simulink model "Tractor_BURGERS_etrailer_v2_1_backup070824"  (R2023a)
settings: Solver=VariableStepAuto  StartTime=0.0  StopTime=tmax  FixedStep=dt  RelTol=1e-3  EnableMultiTasking=on
PreLoadFcn:
  | init_vehicle
  | SIMSCAPE_BE_driveline_etrailer_parameters
StartFcn:
  | tic
StopFcn:
  | toc
  | sim_stop_function
  | Etrailer_Simscape_MBM_plotting
undefined symbols (not defined in the file): brake_input, chassis_length, Diesel_density, Eff, end_val, energyCapacity, etrailer_ON, final_x, final_y, Floor, front_overhang, G_motor, initialSOC, InputSwitch, L_0f, LD, mass_trailer, massload, MaxTrqOut, pose_t0, RPM, sp_t, Std_Regen_Trq, steer_input, steer_path, steer_ratio, steer_sens, throttle_input, tire_param_drive, tire_param_steer, tire_param_trailer, tire_width, Torq, v_0, Voc, Vx, Vx_input, wheelbase, X, Y, Z
libraries: sm_lib x367, nesl_utility x282, fl_lib x20, sdl_lib x2, ee_lib x2, robotalgslib x1, simulink_extras x1, batteryecm_lib x1, BatteryEstimators x1, CommercialVehicleLibrary2G x1
(part 5 of 12)

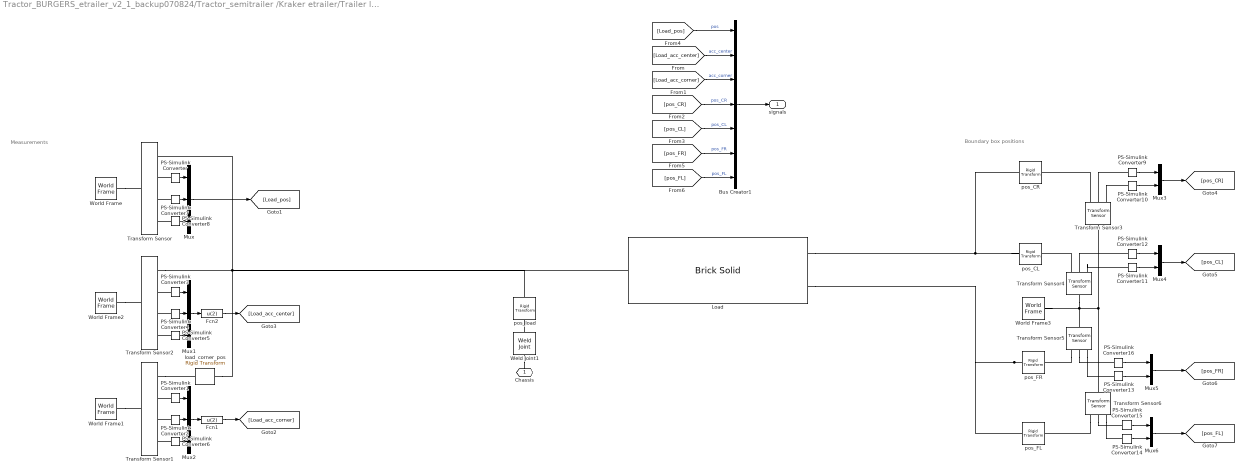
== system Tractor_BURGERS_etrailer_v2_1_backup070824/Tractor_semitrailer /Kraker etrailer/Trailer load front ==
  note: Boundary box positions
  note: Measurements
  Bus Creator1 : BusCreator  Inputs=7
  Fcn1 : Fcn  Expr=u(2)
  Fcn2 : Fcn  Expr=u(2)
  "Load " : sm_lib/Body Elements/Brick Solid  GraphicAmbientColor=[0.15 0.15 0.15 1.0]  BasedOnType=Density  BrickDimensions=[l_load w h]  BrickDimensionsUnits=m  CenterOfMass=[0 0 0]  CenterOfMassUnits=m  GraphicDiffuseColor=[1.0 1.0 0.2]  Density=1000  DensityUnits=kg/m^3  DoExposeReferenceFrame=on  GraphicEmissiveColor=[0.0 0.0 0.0 1.0]  ExportEntireGeometry=off  SerializedFrames=<Frames><Frame><Id>Frame1</Id><Value><Name>Boundary Center</Name><Origin><Source>GeometricFeature</Source><FeatureName>-x surface</FeatureName></Origin><PrimaryAxis><DefinedDirection>+Z</DefinedDirection><Source>ReferenceFrame</Source><SourceDirection>+Z</SourceDirection><FeatureName></FeatureName></PrimaryAxis><SecondaryAxis><DefinedDirection>+X</DefinedDirection><Source>ReferenceFrame</Source><SourceDirection>+X</SourceDirection><FeatureName></FeatureName></SecondaryAxis></Value></Frame><Frame><Id>Frame2</Id><Value><Name>Boundary Front </Name><Origin><Source>GeometricFeature</Source><FeatureName>+x surface</FeatureName></Origin><PrimaryAxis><DefinedDirection>+Z</DefinedDirection><Source>ReferenceFrame</Source><SourceDirection>+Z</SourceDirection><FeatureName></FeatureName></PrimaryAxis><SecondaryAxis><DefinedDirection>+X</DefinedDirection><Source>ReferenceFrame</Source><SourceDirection>+X</SourceDirection><FeatureName></FeatureName></SecondaryAxis></Value></Frame></Frames>  MarkerShape=Sphere  MarkerSize=10  GraphicType=FromGeometry  InertiaType=Custom  Mass=mass_load  MassUnits=kg  MomentsOfInertia=[Ixx Iyy Izz]  MomentsOfInertiaUnits=kg*m^2  GraphicOpacity=0.5  ProductsOfInertia=[0 0 0]  ProductsOfInertiaUnits=kg*m^2  GraphicShininess=75  GraphicSpecularColor=[0.5 0.5 0.5 1.0]  GraphicVisPropType=SimpleVisualProperties
  Mux : Mux  Inputs=3
  Mux1 : Mux  Inputs=3
  Mux2 : Mux  Inputs=3
  Mux{3..6} (4 alike) : Mux  Inputs=2
  PS-Simulink Converter{,7..16} (11 alike) : nesl_utility/PS-Simulink Converter  PhysicalDomain=network_engine_domain  SubClassName=ps_output  LeftPortType=input  RightPortType=output  PseudoPeriodic=off  Frequencies=[]  VectorFormat=1-D array  Unit=inherit  AffineConversion=off
  PS-Simulink Converter{1..6} (6 alike) : nesl_utility/PS-Simulink Converter  PhysicalDomain=network_engine_domain  SubClassName=ps_output  LeftPortType=input  RightPortType=output  PseudoPeriodic=off  Frequencies=[]  VectorFormat=1-D array  Unit=m/s^2  AffineConversion=off
  Transform Sensor : sm_lib/Frames and Transforms/Transform Sensor  MeasurementFrame=World  RotationSequence=XYX  SenseAngle=off  SenseAxis=off  SenseQ=off  SenseR=off  SenseRotationSequence=off  SenseOmegaX=off  SenseOmegaY=off  SenseOmegaZ=off  SenseQDot=off  SenseRDot=off  SenseRotationSequenceDot=off  SenseAlphaX=off  SenseAlphaY=off  SenseAlphaZ=off  SenseQDDot=off  SenseRDDot=off  SenseX=on  SenseY=on  SenseZ=on  SenseRad=off  SenseAzim=off  SenseDist=off  SenseInc=off  SenseXDot=off  SenseYDot=off  SenseZDot=off  SenseRadDot=off  SenseAzimDot=off  SenseDistDot=off  SenseIncDot=off  SenseXDDot=off  SenseYDDot=off  SenseZDDot=off  SenseRadDDot=off  SenseAzimDDot=off  SenseDistDDot=off  SenseIncDDot=off
  Transform Sensor1 : sm_lib/Frames and Transforms/Transform Sensor  MeasurementFrame=NonRotatingFollower  RotationSequence=XYX  SenseAngle=off  SenseAxis=off  SenseQ=off  SenseR=off  SenseRotationSequence=off  SenseOmegaX=off  SenseOmegaY=off  SenseOmegaZ=off  SenseQDot=off  SenseRDot=off  SenseRotationSequenceDot=off  SenseAlphaX=off  SenseAlphaY=off  SenseAlphaZ=off  SenseQDDot=off  SenseRDDot=off  SenseX=off  SenseY=off  SenseZ=off  SenseRad=off  SenseAzim=off  SenseDist=off  SenseInc=off  SenseXDot=off  SenseYDot=off  SenseZDot=off  SenseRadDot=off  SenseAzimDot=off  SenseDistDot=off  SenseIncDot=off  SenseXDDot=on  SenseYDDot=on  SenseZDDot=on  SenseRadDDot=off  SenseAzimDDot=off  SenseDistDDot=off  SenseIncDDot=off
  Transform Sensor2 : sm_lib/Frames and Transforms/Transform Sensor  MeasurementFrame=NonRotatingFollower  RotationSequence=XYX  SenseAngle=off  SenseAxis=off  SenseQ=off  SenseR=off  SenseRotationSequence=off  SenseOmegaX=off  SenseOmegaY=off  SenseOmegaZ=off  SenseQDot=off  SenseRDot=off  SenseRotationSequenceDot=off  SenseAlphaX=off  SenseAlphaY=off  SenseAlphaZ=off  SenseQDDot=off  SenseRDDot=off  SenseX=off  SenseY=off  SenseZ=off  SenseRad=off  SenseAzim=off  SenseDist=off  SenseInc=off  SenseXDot=off  SenseYDot=off  SenseZDot=off  SenseRadDot=off  SenseAzimDot=off  SenseDistDot=off  SenseIncDot=off  SenseXDDot=on  SenseYDDot=on  SenseZDDot=on  SenseRadDDot=off  SenseAzimDDot=off  SenseDistDDot=off  SenseIncDDot=off
  Transform Sensor{3..6} (4 alike) : sm_lib/Frames and Transforms/Transform Sensor  MeasurementFrame=World  RotationSequence=XYX  SenseAngle=off  SenseAxis=off  SenseQ=off  SenseR=off  SenseRotationSequence=off  SenseOmegaX=off  SenseOmegaY=off  SenseOmegaZ=off  SenseQDot=off  SenseRDot=off  SenseRotationSequenceDot=off  SenseAlphaX=off  SenseAlphaY=off  SenseAlphaZ=off  SenseQDDot=off  SenseRDDot=off  SenseX=on  SenseY=on  SenseZ=off  SenseRad=off  SenseAzim=off  SenseDist=off  SenseInc=off  SenseXDot=off  SenseYDot=off  SenseZDot=off  SenseRadDot=off  SenseAzimDot=off  SenseDistDot=off  SenseIncDot=off  SenseXDDot=off  SenseYDDot=off  SenseZDDot=off  SenseRadDDot=off  SenseAzimDDot=off  SenseDistDDot=off  SenseIncDDot=off
  Weld Joint1 : sm_lib/Joints/Weld Joint  JointMode=Normal  SenseConstraintForce=off  SenseConstraintForceX=off  SenseConstraintForceY=off  SenseConstraintForceZ=off  SenseConstraintTorque=off  SenseConstraintTorqueX=off  SenseConstraintTorqueY=off  SenseConstraintTorqueZ=off  SenseTotalForce=off  SenseTotalForceX=off  SenseTotalForceY=off  SenseTotalForceZ=off  SenseTotalTorque=off  SenseTotalTorqueX=off  SenseTotalTorqueY=off  SenseTotalTorqueZ=off  CompositeWrenchDir=FollowerOnBase  CompositeWrenchFrame=BaseFrame
  World Frame{,1..3} (4 alike) : sm_lib/Frames and Transforms/World Frame
  load_corner_pos : sm_lib/Frames and Transforms/Rigid Transform  TranslationMethod=Cartesian  TranslationStandardOffset=0  TranslationStandardOffsetUnits=m  TranslationStandardAxis=+Z  TranslationCartesianOffset=[(-0.5*l_load) 0 0]  TranslationCartesianOffsetUnits=m  TranslationROffset=0  TranslationROffsetUnits=m  TranslationZOffset=0  TranslationZOffsetUnits=m  TranslationThetaOffset=0  TranslationThetaOffsetUnits=deg  RotationMethod=None  RotationAngleUnits=deg  RotationStandardAxis=+Z  RotationAngle=0.0  RotationArbitraryAxis=[0 0 1]  FollAlignAxisA=+X  BaseAlignAxisA=+Y  FollAlignAxisB=+Y  BaseAlignAxisB=+Z  RotationSequenceAxes=FollowerAxes  RotationSequence=XYX  RotationSequenceAngles=[0 0 0]  RotationSequenceAnglesUnits=deg  RotationMatrix=[1 0 0; 0 1 0; 0 0 1]  Quaternion=[1 0 0 0]
  pos_CL : sm_lib/Frames and Transforms/Rigid Transform  TranslationMethod=Cartesian  TranslationStandardOffset=0  TranslationStandardOffsetUnits=m  TranslationStandardAxis=+Z  TranslationCartesianOffset=[0 w/2 -h/2]  TranslationCartesianOffsetUnits=m  TranslationROffset=0  TranslationROffsetUnits=m  TranslationZOffset=0  TranslationZOffsetUnits=m  TranslationThetaOffset=0  TranslationThetaOffsetUnits=deg  RotationMethod=None  RotationAngleUnits=deg  RotationStandardAxis=+Z  RotationAngle=0.0  RotationArbitraryAxis=[0 0 1]  FollAlignAxisA=+X  BaseAlignAxisA=+Y  FollAlignAxisB=+Y  BaseAlignAxisB=+Z  RotationSequenceAxes=FollowerAxes  RotationSequence=XYX  RotationSequenceAngles=[0 0 0]  RotationSequenceAnglesUnits=deg  RotationMatrix=[1 0 0; 0 1 0; 0 0 1]  Quaternion=[1 0 0 0]
  pos_CR : sm_lib/Frames and Transforms/Rigid Transform  TranslationMethod=Cartesian  TranslationStandardOffset=0  TranslationStandardOffsetUnits=m  TranslationStandardAxis=+Z  TranslationCartesianOffset=[0 -w/2 -h/2]  TranslationCartesianOffsetUnits=m  TranslationROffset=0  TranslationROffsetUnits=m  TranslationZOffset=0  TranslationZOffsetUnits=m  TranslationThetaOffset=0  TranslationThetaOffsetUnits=deg  RotationMethod=None  RotationAngleUnits=deg  RotationStandardAxis=+Z  RotationAngle=0.0  RotationArbitraryAxis=[0 0 1]  FollAlignAxisA=+X  BaseAlignAxisA=+Y  FollAlignAxisB=+Y  BaseAlignAxisB=+Z  RotationSequenceAxes=FollowerAxes  RotationSequence=XYX  RotationSequenceAngles=[0 0 0]  RotationSequenceAnglesUnits=deg  RotationMatrix=[1 0 0; 0 1 0; 0 0 1]  Quaternion=[1 0 0 0]
  pos_FL : sm_lib/Frames and Transforms/Rigid Transform  TranslationMethod=Cartesian  TranslationStandardOffset=0  TranslationStandardOffsetUnits=m  TranslationStandardAxis=+Z  TranslationCartesianOffset=[0 w/2 -h/2]  TranslationCartesianOffsetUnits=m  TranslationROffset=0  TranslationROffsetUnits=m  TranslationZOffset=0  TranslationZOffsetUnits=m  TranslationThetaOffset=0  TranslationThetaOffsetUnits=deg  RotationMethod=None  RotationAngleUnits=deg  RotationStandardAxis=+Z  RotationAngle=0.0  RotationArbitraryAxis=[0 0 1]  FollAlignAxisA=+X  BaseAlignAxisA=+Y  FollAlignAxisB=+Y  BaseAlignAxisB=+Z  RotationSequenceAxes=FollowerAxes  RotationSequence=XYX  RotationSequenceAngles=[0 0 0]  RotationSequenceAnglesUnits=deg  RotationMatrix=[1 0 0; 0 1 0; 0 0 1]  Quaternion=[1 0 0 0]
  pos_FR : sm_lib/Frames and Transforms/Rigid Transform  TranslationMethod=Cartesian  TranslationStandardOffset=0  TranslationStandardOffsetUnits=m  TranslationStandardAxis=+Z  TranslationCartesianOffset=[0 -w/2 -h/2]  TranslationCartesianOffsetUnits=m  TranslationROffset=0  TranslationROffsetUnits=m  TranslationZOffset=0  TranslationZOffsetUnits=m  TranslationThetaOffset=0  TranslationThetaOffsetUnits=deg  RotationMethod=None  RotationAngleUnits=deg  RotationStandardAxis=+Z  RotationAngle=0.0  RotationArbitraryAxis=[0 0 1]  FollAlignAxisA=+X  BaseAlignAxisA=+Y  FollAlignAxisB=+Y  BaseAlignAxisB=+Z  RotationSequenceAxes=FollowerAxes  RotationSequence=XYX  RotationSequenceAngles=[0 0 0]  RotationSequenceAnglesUnits=deg  RotationMatrix=[1 0 0; 0 1 0; 0 0 1]  Quaternion=[1 0 0 0]
  pos_load : sm_lib/Frames and Transforms/Rigid Transform  TranslationMethod=Cartesian  TranslationStandardOffset=0  TranslationStandardOffsetUnits=m  TranslationStandardAxis=+Z  TranslationCartesianOffset=[-xcg1+xload 0 zcg+0.1]  TranslationCartesianOffsetUnits=m  TranslationROffset=0  TranslationROffsetUnits=m  TranslationZOffset=0  TranslationZOffsetUnits=m  TranslationThetaOffset=0  TranslationThetaOffsetUnits=deg  RotationMethod=None  RotationAngleUnits=deg  RotationStandardAxis=+Z  RotationAngle=0.0  RotationArbitraryAxis=[0 0 1]  FollAlignAxisA=+X  BaseAlignAxisA=+Y  FollAlignAxisB=+Y  BaseAlignAxisB=+Z  RotationSequenceAxes=FollowerAxes  RotationSequence=XYX  RotationSequenceAngles=[0 0 0]  RotationSequenceAnglesUnits=deg  RotationMatrix=[1 0 0; 0 1 0; 0 0 1]  Quaternion=[1 0 0 0]
  Chassis : PMIOPort  Side=Left
  signals : Outport
  wires:
  [Load_acc_corner] -> Bus Creator1/3  "acc_corner"
  PS-Simulink Converter1/1 -> Mux2/1
  Mux2/1 -> Fcn1/1
  PS-Simulink Converter6/1 -> Mux2/3
  Fcn1/1 -> [Load_acc_corner]
  PS-Simulink Converter2/1 -> Mux2/2
  [Load_pos] -> Bus Creator1/1  "pos"
  Bus Creator1/1 -> signals/1
  [Load_acc_center] -> Bus Creator1/2  "acc_center"
  PS-Simulink Converter4/1 -> Mux1/2
  Fcn2/1 -> [Load_acc_center]
  PS-Simulink Converter5/1 -> Mux1/3
  Mux/1 -> [Load_pos]
  Mux1/1 -> Fcn2/1
  PS-Simulink Converter3/1 -> Mux1/1
  PS-Simulink Converter8/1 -> Mux/3
  PS-Simulink Converter/1 -> Mux/1
  PS-Simulink Converter7/1 -> Mux/2
  PS-Simulink Converter9/1 -> Mux3/1
  PS-Simulink Converter10/1 -> Mux3/2
  PS-Simulink Converter11/1 -> Mux4/2
  PS-Simulink Converter12/1 -> Mux4/1
  Mux3/1 -> [pos_CR]
  Mux4/1 -> [pos_CL]
  Mux5/1 -> [pos_FR]
  PS-Simulink Converter14/1 -> Mux6/2
  PS-Simulink Converter15/1 -> Mux6/1
  Mux6/1 -> [pos_FL]
  PS-Simulink Converter16/1 -> Mux5/1
  PS-Simulink Converter13/1 -> Mux5/2
  [pos_CR] -> Bus Creator1/4  "pos_CR"
  [pos_FR] -> Bus Creator1/6  "pos_FR"
  [pos_CL] -> Bus Creator1/5  "pos_CL"
  [pos_FL] -> Bus Creator1/7  "pos_FL"
  connections:
  Transform Sensor1/RConn1 -- load_corner_pos/RConn1
  PS-Simulink Converter2/LConn1 -- Transform Sensor1/RConn3
  PS-Simulink Converter1/LConn1 -- Transform Sensor1/RConn2
  PS-Simulink Converter6/LConn1 -- Transform Sensor1/RConn4
  World Frame1/RConn1 -- Transform Sensor1/LConn1
  Weld Joint1/LConn1 -- Chassis/RConn1
  Weld Joint1/RConn1 -- pos_load/LConn1
  World Frame2/RConn1 -- Transform Sensor2/LConn1
  PS-Simulink Converter/LConn1 -- Transform Sensor/RConn2
  PS-Simulink Converter5/LConn1 -- Transform Sensor2/RConn4
  PS-Simulink Converter3/LConn1 -- Transform Sensor2/RConn2
  World Frame/RConn1 -- Transform Sensor/LConn1
  PS-Simulink Converter4/LConn1 -- Transform Sensor2/RConn3
  PS-Simulink Converter7/LConn1 -- Transform Sensor/RConn3
  PS-Simulink Converter8/LConn1 -- Transform Sensor/RConn4
  load_corner_pos/LConn1 -- Transform Sensor/RConn1 -- Transform Sensor2/RConn1 -- pos_load/RConn1 -- "Load "/RConn1
  pos_CL/LConn1 -- pos_CR/LConn1 -- "Load "/LConn1
  pos_FR/LConn1 -- "Load "/LConn2 -- pos_FL/LConn1
  World Frame3/RConn1 -- Transform Sensor5/LConn1 -- Transform Sensor4/LConn1 -- Transform Sensor3/LConn1 -- Transform Sensor6/LConn1
  Transform Sensor3/RConn1 -- pos_CR/RConn1
  Transform Sensor3/RConn2 -- PS-Simulink Converter9/LConn1
  Transform Sensor3/RConn3 -- PS-Simulink Converter10/LConn1
  Transform Sensor4/RConn1 -- pos_CL/RConn1
  Transform Sensor4/RConn2 -- PS-Simulink Converter12/LConn1
  Transform Sensor4/RConn3 -- PS-Simulink Converter11/LConn1
  Transform Sensor6/RConn2 -- PS-Simulink Converter15/LConn1
  Transform Sensor5/RConn3 -- PS-Simulink Converter13/LConn1
  Transform Sensor6/RConn1 -- pos_FL/RConn1
  Transform Sensor5/RConn2 -- PS-Simulink Converter16/LConn1
  Transform Sensor6/RConn3 -- PS-Simulink Converter14/LConn1
  Transform Sensor5/RConn1 -- pos_FR/RConn1

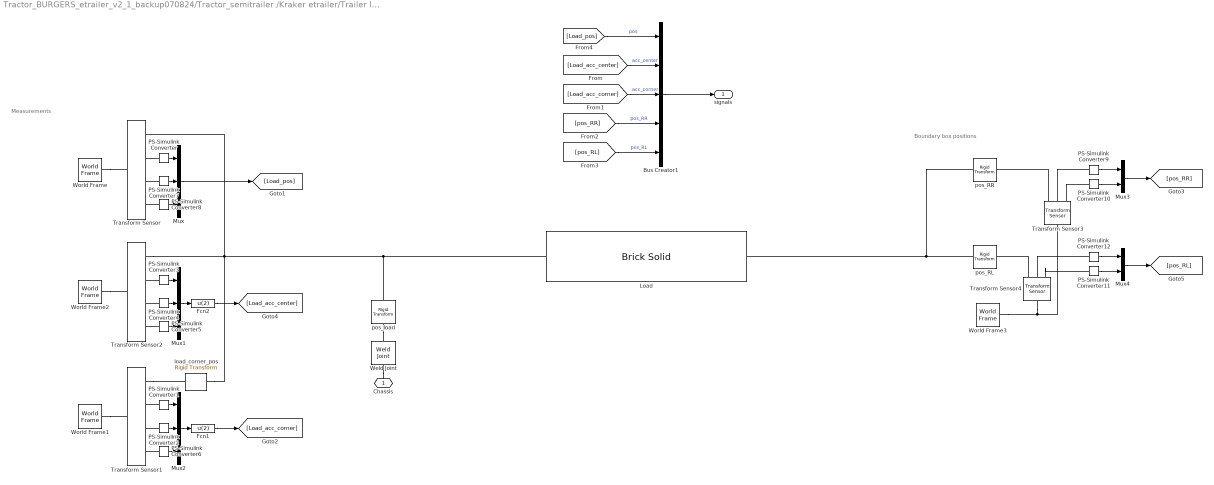
== system Tractor_BURGERS_etrailer_v2_1_backup070824/Tractor_semitrailer /Kraker etrailer/Trailer load rear ==
  note: Measurements
  note: Boundary box positions
  Bus Creator1 : BusCreator  Inputs=5
  Fcn1 : Fcn  Expr=u(2)
  Fcn2 : Fcn  Expr=u(2)
  "Load " : sm_lib/Body Elements/Brick Solid  GraphicAmbientColor=[0.15 0.15 0.15 1.0]  BasedOnType=Density  BrickDimensions=[l_load2 w h]  BrickDimensionsUnits=m  CenterOfMass=[0 0 0]  CenterOfMassUnits=m  GraphicDiffuseColor=[1.0 1.0 0.2]  Density=1000  DensityUnits=kg/m^3  DoExposeReferenceFrame=on  GraphicEmissiveColor=[0.0 0.0 0.0 1.0]  ExportEntireGeometry=off  SerializedFrames=<Frames><Frame><Id>Frame1</Id><Value><Name>Boundary rear </Name><Origin><Source>GeometricFeature</Source><FeatureName>-x surface</FeatureName></Origin><PrimaryAxis><DefinedDirection>+Z</DefinedDirection><Source>ReferenceFrame</Source><SourceDirection>+Z</SourceDirection><FeatureName></FeatureName></PrimaryAxis><SecondaryAxis><DefinedDirection>+X</DefinedDirection><Source>ReferenceFrame</Source><SourceDirection>+X</SourceDirection><FeatureName></FeatureName></SecondaryAxis></Value></Frame></Frames>  MarkerShape=Sphere  MarkerSize=10  GraphicType=FromGeometry  InertiaType=Custom  Mass=mass_load  MassUnits=kg  MomentsOfInertia=[Ixx Iyy Izz]  MomentsOfInertiaUnits=kg*m^2  GraphicOpacity=0.5  ProductsOfInertia=[0 0 0]  ProductsOfInertiaUnits=kg*m^2  GraphicShininess=75  GraphicSpecularColor=[0.5 0.5 0.5 1.0]  GraphicVisPropType=SimpleVisualProperties
  Mux : Mux  Inputs=3
  Mux1 : Mux  Inputs=3
  Mux2 : Mux  Inputs=3
  Mux3 : Mux  Inputs=2
  Mux4 : Mux  Inputs=2
  PS-Simulink Converter{,7..12} (7 alike) : nesl_utility/PS-Simulink Converter  PhysicalDomain=network_engine_domain  SubClassName=ps_output  LeftPortType=input  RightPortType=output  PseudoPeriodic=off  Frequencies=[]  VectorFormat=1-D array  Unit=inherit  AffineConversion=off
  PS-Simulink Converter{1..6} (6 alike) : nesl_utility/PS-Simulink Converter  PhysicalDomain=network_engine_domain  SubClassName=ps_output  LeftPortType=input  RightPortType=output  PseudoPeriodic=off  Frequencies=[]  VectorFormat=1-D array  Unit=m/s^2  AffineConversion=off
  Transform Sensor : sm_lib/Frames and Transforms/Transform Sensor  MeasurementFrame=World  RotationSequence=XYX  SenseAngle=off  SenseAxis=off  SenseQ=off  SenseR=off  SenseRotationSequence=off  SenseOmegaX=off  SenseOmegaY=off  SenseOmegaZ=off  SenseQDot=off  SenseRDot=off  SenseRotationSequenceDot=off  SenseAlphaX=off  SenseAlphaY=off  SenseAlphaZ=off  SenseQDDot=off  SenseRDDot=off  SenseX=on  SenseY=on  SenseZ=on  SenseRad=off  SenseAzim=off  SenseDist=off  SenseInc=off  SenseXDot=off  SenseYDot=off  SenseZDot=off  SenseRadDot=off  SenseAzimDot=off  SenseDistDot=off  SenseIncDot=off  SenseXDDot=off  SenseYDDot=off  SenseZDDot=off  SenseRadDDot=off  SenseAzimDDot=off  SenseDistDDot=off  SenseIncDDot=off
  Transform Sensor1 : sm_lib/Frames and Transforms/Transform Sensor  MeasurementFrame=NonRotatingFollower  RotationSequence=XYX  SenseAngle=off  SenseAxis=off  SenseQ=off  SenseR=off  SenseRotationSequence=off  SenseOmegaX=off  SenseOmegaY=off  SenseOmegaZ=off  SenseQDot=off  SenseRDot=off  SenseRotationSequenceDot=off  SenseAlphaX=off  SenseAlphaY=off  SenseAlphaZ=off  SenseQDDot=off  SenseRDDot=off  SenseX=off  SenseY=off  SenseZ=off  SenseRad=off  SenseAzim=off  SenseDist=off  SenseInc=off  SenseXDot=off  SenseYDot=off  SenseZDot=off  SenseRadDot=off  SenseAzimDot=off  SenseDistDot=off  SenseIncDot=off  SenseXDDot=on  SenseYDDot=on  SenseZDDot=on  SenseRadDDot=off  SenseAzimDDot=off  SenseDistDDot=off  SenseIncDDot=off
  Transform Sensor2 : sm_lib/Frames and Transforms/Transform Sensor  MeasurementFrame=NonRotatingFollower  RotationSequence=XYX  SenseAngle=off  SenseAxis=off  SenseQ=off  SenseR=off  SenseRotationSequence=off  SenseOmegaX=off  SenseOmegaY=off  SenseOmegaZ=off  SenseQDot=off  SenseRDot=off  SenseRotationSequenceDot=off  SenseAlphaX=off  SenseAlphaY=off  SenseAlphaZ=off  SenseQDDot=off  SenseRDDot=off  SenseX=off  SenseY=off  SenseZ=off  SenseRad=off  SenseAzim=off  SenseDist=off  SenseInc=off  SenseXDot=off  SenseYDot=off  SenseZDot=off  SenseRadDot=off  SenseAzimDot=off  SenseDistDot=off  SenseIncDot=off  SenseXDDot=on  SenseYDDot=on  SenseZDDot=on  SenseRadDDot=off  SenseAzimDDot=off  SenseDistDDot=off  SenseIncDDot=off
  Transform Sensor3 : sm_lib/Frames and Transforms/Transform Sensor  MeasurementFrame=World  RotationSequence=XYX  SenseAngle=off  SenseAxis=off  SenseQ=off  SenseR=off  SenseRotationSequence=off  SenseOmegaX=off  SenseOmegaY=off  SenseOmegaZ=off  SenseQDot=off  SenseRDot=off  SenseRotationSequenceDot=off  SenseAlphaX=off  SenseAlphaY=off  SenseAlphaZ=off  SenseQDDot=off  SenseRDDot=off  SenseX=on  SenseY=on  SenseZ=off  SenseRad=off  SenseAzim=off  SenseDist=off  SenseInc=off  SenseXDot=off  SenseYDot=off  SenseZDot=off  SenseRadDot=off  SenseAzimDot=off  SenseDistDot=off  SenseIncDot=off  SenseXDDot=off  SenseYDDot=off  SenseZDDot=off  SenseRadDDot=off  SenseAzimDDot=off  SenseDistDDot=off  SenseIncDDot=off
  Transform Sensor4 : sm_lib/Frames and Transforms/Transform Sensor  MeasurementFrame=World  RotationSequence=XYX  SenseAngle=off  SenseAxis=off  SenseQ=off  SenseR=off  SenseRotationSequence=off  SenseOmegaX=off  SenseOmegaY=off  SenseOmegaZ=off  SenseQDot=off  SenseRDot=off  SenseRotationSequenceDot=off  SenseAlphaX=off  SenseAlphaY=off  SenseAlphaZ=off  SenseQDDot=off  SenseRDDot=off  SenseX=on  SenseY=on  SenseZ=off  SenseRad=off  SenseAzim=off  SenseDist=off  SenseInc=off  SenseXDot=off  SenseYDot=off  SenseZDot=off  SenseRadDot=off  SenseAzimDot=off  SenseDistDot=off  SenseIncDot=off  SenseXDDot=off  SenseYDDot=off  SenseZDDot=off  SenseRadDDot=off  SenseAzimDDot=off  SenseDistDDot=off  SenseIncDDot=off
  Weld Joint : sm_lib/Joints/Weld Joint  JointMode=Normal  SenseConstraintForce=off  SenseConstraintForceX=off  SenseConstraintForceY=off  SenseConstraintForceZ=off  SenseConstraintTorque=off  SenseConstraintTorqueX=off  SenseConstraintTorqueY=off  SenseConstraintTorqueZ=off  SenseTotalForce=off  SenseTotalForceX=off  SenseTotalForceY=off  SenseTotalForceZ=off  SenseTotalTorque=off  SenseTotalTorqueX=off  SenseTotalTorqueY=off  SenseTotalTorqueZ=off  CompositeWrenchDir=FollowerOnBase  CompositeWrenchFrame=BaseFrame
  World Frame{,1..3} (4 alike) : sm_lib/Frames and Transforms/World Frame
  load_corner_pos : sm_lib/Frames and Transforms/Rigid Transform  TranslationMethod=Cartesian  TranslationStandardOffset=0  TranslationStandardOffsetUnits=m  TranslationStandardAxis=+Z  TranslationCartesianOffset=[(-0.5*l_load) 0 0]  TranslationCartesianOffsetUnits=m  TranslationROffset=0  TranslationROffsetUnits=m  TranslationZOffset=0  TranslationZOffsetUnits=m  TranslationThetaOffset=0  TranslationThetaOffsetUnits=deg  RotationMethod=None  RotationAngleUnits=deg  RotationStandardAxis=+Z  RotationAngle=0.0  RotationArbitraryAxis=[0 0 1]  FollAlignAxisA=+X  BaseAlignAxisA=+Y  FollAlignAxisB=+Y  BaseAlignAxisB=+Z  RotationSequenceAxes=FollowerAxes  RotationSequence=XYX  RotationSequenceAngles=[0 0 0]  RotationSequenceAnglesUnits=deg  RotationMatrix=[1 0 0; 0 1 0; 0 0 1]  Quaternion=[1 0 0 0]
  pos_RL : sm_lib/Frames and Transforms/Rigid Transform  TranslationMethod=Cartesian  TranslationStandardOffset=0  TranslationStandardOffsetUnits=m  TranslationStandardAxis=+Z  TranslationCartesianOffset=[0 w/2 -h/2]  TranslationCartesianOffsetUnits=m  TranslationROffset=0  TranslationROffsetUnits=m  TranslationZOffset=0  TranslationZOffsetUnits=m  TranslationThetaOffset=0  TranslationThetaOffsetUnits=deg  RotationMethod=None  RotationAngleUnits=deg  RotationStandardAxis=+Z  RotationAngle=0.0  RotationArbitraryAxis=[0 0 1]  FollAlignAxisA=+X  BaseAlignAxisA=+Y  FollAlignAxisB=+Y  BaseAlignAxisB=+Z  RotationSequenceAxes=FollowerAxes  RotationSequence=XYX  RotationSequenceAngles=[0 0 0]  RotationSequenceAnglesUnits=deg  RotationMatrix=[1 0 0; 0 1 0; 0 0 1]  Quaternion=[1 0 0 0]
  pos_RR : sm_lib/Frames and Transforms/Rigid Transform  TranslationMethod=Cartesian  TranslationStandardOffset=0  TranslationStandardOffsetUnits=m  TranslationStandardAxis=+Z  TranslationCartesianOffset=[0 -w/2 -h/2]  TranslationCartesianOffsetUnits=m  TranslationROffset=0  TranslationROffsetUnits=m  TranslationZOffset=0  TranslationZOffsetUnits=m  TranslationThetaOffset=0  TranslationThetaOffsetUnits=deg  RotationMethod=None  RotationAngleUnits=deg  RotationStandardAxis=+Z  RotationAngle=0.0  RotationArbitraryAxis=[0 0 1]  FollAlignAxisA=+X  BaseAlignAxisA=+Y  FollAlignAxisB=+Y  BaseAlignAxisB=+Z  RotationSequenceAxes=FollowerAxes  RotationSequence=XYX  RotationSequenceAngles=[0 0 0]  RotationSequenceAnglesUnits=deg  RotationMatrix=[1 0 0; 0 1 0; 0 0 1]  Quaternion=[1 0 0 0]
  pos_load : sm_lib/Frames and Transforms/Rigid Transform  TranslationMethod=Cartesian  TranslationStandardOffset=0  TranslationStandardOffsetUnits=m  TranslationStandardAxis=+Z  TranslationCartesianOffset=[-xcg2+xload 0 zcg+0.1]  TranslationCartesianOffsetUnits=m  TranslationROffset=0  TranslationROffsetUnits=m  TranslationZOffset=0  TranslationZOffsetUnits=m  TranslationThetaOffset=0  TranslationThetaOffsetUnits=deg  RotationMethod=None  RotationAngleUnits=deg  RotationStandardAxis=+Z  RotationAngle=0.0  RotationArbitraryAxis=[0 0 1]  FollAlignAxisA=+X  BaseAlignAxisA=+Y  FollAlignAxisB=+Y  BaseAlignAxisB=+Z  RotationSequenceAxes=FollowerAxes  RotationSequence=XYX  RotationSequenceAngles=[0 0 0]  RotationSequenceAnglesUnits=deg  RotationMatrix=[1 0 0; 0 1 0; 0 0 1]  Quaternion=[1 0 0 0]
  Chassis : PMIOPort  Side=Left
  signals : Outport
  wires:
  [Load_acc_corner] -> Bus Creator1/3  "acc_corner"
  Fcn1/1 -> [Load_acc_corner]
  Mux2/1 -> Fcn1/1
  PS-Simulink Converter6/1 -> Mux2/3
  PS-Simulink Converter1/1 -> Mux2/1
  PS-Simulink Converter2/1 -> Mux2/2
  [Load_pos] -> Bus Creator1/1  "pos"
  Bus Creator1/1 -> signals/1
  [Load_acc_center] -> Bus Creator1/2  "acc_center"
  PS-Simulink Converter4/1 -> Mux1/2
  Fcn2/1 -> [Load_acc_center]
  PS-Simulink Converter5/1 -> Mux1/3
  Mux/1 -> [Load_pos]
  Mux1/1 -> Fcn2/1
  PS-Simulink Converter3/1 -> Mux1/1
  PS-Simulink Converter8/1 -> Mux/3
  PS-Simulink Converter/1 -> Mux/1
  PS-Simulink Converter7/1 -> Mux/2
  PS-Simulink Converter10/1 -> Mux3/2
  PS-Simulink Converter9/1 -> Mux3/1
  Mux3/1 -> [pos_RR]
  PS-Simulink Converter11/1 -> Mux4/2
  PS-Simulink Converter12/1 -> Mux4/1
  Mux4/1 -> [pos_RL]
  [pos_RR] -> Bus Creator1/4  "pos_RR"
  [pos_RL] -> Bus Creator1/5  "pos_RL"
  connections:
  PS-Simulink Converter2/LConn1 -- Transform Sensor1/RConn3
  PS-Simulink Converter1/LConn1 -- Transform Sensor1/RConn2
  Transform Sensor1/RConn1 -- load_corner_pos/RConn1
  World Frame1/RConn1 -- Transform Sensor1/LConn1
  PS-Simulink Converter6/LConn1 -- Transform Sensor1/RConn4
  Weld Joint/LConn1 -- Chassis/RConn1
  pos_load/LConn1 -- Weld Joint/RConn1
  World Frame2/RConn1 -- Transform Sensor2/LConn1
  PS-Simulink Converter/LConn1 -- Transform Sensor/RConn2
  PS-Simulink Converter5/LConn1 -- Transform Sensor2/RConn4
  PS-Simulink Converter3/LConn1 -- Transform Sensor2/RConn2
  World Frame/RConn1 -- Transform Sensor/LConn1
  PS-Simulink Converter4/LConn1 -- Transform Sensor2/RConn3
  PS-Simulink Converter7/LConn1 -- Transform Sensor/RConn3
  PS-Simulink Converter8/LConn1 -- Transform Sensor/RConn4
  load_corner_pos/LConn1 -- pos_load/RConn1 -- "Load "/RConn1 -- Transform Sensor2/RConn1 -- Transform Sensor/RConn1
  World Frame3/RConn1 -- Transform Sensor4/LConn1 -- Transform Sensor3/LConn1
  pos_RL/LConn1 -- "Load "/LConn1 -- pos_RR/LConn1
  Transform Sensor3/RConn1 -- pos_RR/RConn1
  Transform Sensor4/RConn3 -- PS-Simulink Converter11/LConn1
  Transform Sensor4/RConn2 -- PS-Simulink Converter12/LConn1
  Transform Sensor4/RConn1 -- pos_RL/RConn1
  Transform Sensor3/RConn3 -- PS-Simulink Converter10/LConn1
  Transform Sensor3/RConn2 -- PS-Simulink Converter9/LConn1

== system Tractor_BURGERS_etrailer_v2_1_backup070824/Tractor_semitrailer /Kraker etrailer/Trailer_torsion ==
  Align_Torsion joint : sm_lib/Frames and Transforms/Rigid Transform  TranslationMethod=None  TranslationStandardOffset=0  TranslationStandardOffsetUnits=m  TranslationStandardAxis=+Z  TranslationCartesianOffset=[-0.5*l 0 0]  TranslationCartesianOffsetUnits=m  TranslationROffset=0  TranslationROffsetUnits=m  TranslationZOffset=0  TranslationZOffsetUnits=m  TranslationThetaOffset=0  TranslationThetaOffsetUnits=deg  RotationMethod=AlignedAxes  RotationAngleUnits=deg  RotationStandardAxis=+Z  RotationAngle=0.0  RotationArbitraryAxis=[0 0 1]  FollAlignAxisA=+X  BaseAlignAxisA=+Z  FollAlignAxisB=+Y  BaseAlignAxisB=+Y  RotationSequenceAxes=FollowerAxes  RotationSequence=XYX  RotationSequenceAngles=[0 0 0]  RotationSequenceAnglesUnits=deg  RotationMatrix=[1 0 0; 0 1 0; 0 0 1]  Quaternion=[1 0 0 0]
  Bus Creator1 : BusCreator  Inputs=3
  Chassis rear pos : sm_lib/Frames and Transforms/Rigid Transform  TranslationMethod=Cartesian  TranslationStandardOffset=2.02-0.08  TranslationStandardOffsetUnits=m  TranslationStandardAxis=-X  TranslationCartesianOffset=[-xrev1+xcg2 0 0]  TranslationCartesianOffsetUnits=m  TranslationROffset=0  TranslationROffsetUnits=m  TranslationZOffset=0  TranslationZOffsetUnits=m  TranslationThetaOffset=0  TranslationThetaOffsetUnits=deg  RotationMethod=None  RotationAngleUnits=deg  RotationStandardAxis=+Z  RotationAngle=0.0  RotationArbitraryAxis=[0 0 1]  FollAlignAxisA=+X  BaseAlignAxisA=+Y  FollAlignAxisB=+Y  BaseAlignAxisB=+Z  RotationSequenceAxes=FollowerAxes  RotationSequence=XYX  RotationSequenceAngles=[0 0 0]  RotationSequenceAnglesUnits=deg  RotationMatrix=[1 0 0; 0 1 0; 0 0 1]  Quaternion=[1 0 0 0]
  PS-Simulink Converter - in rad : nesl_utility/PS-Simulink Converter  PhysicalDomain=network_engine_domain  SubClassName=ps_output  LeftPortType=input  RightPortType=output  PseudoPeriodic=off  Frequencies=[]  VectorFormat=1-D array  Unit=rad  AffineConversion=off
  PS-Simulink Converter4 : nesl_utility/PS-Simulink Converter  PhysicalDomain=network_engine_domain  SubClassName=ps_output  LeftPortType=input  RightPortType=output  PseudoPeriodic=off  Frequencies=[]  VectorFormat=1-D array  Unit=1  AffineConversion=off
  Realign_Torsion joint : sm_lib/Frames and Transforms/Rigid Transform  TranslationMethod=None  TranslationStandardOffset=0  TranslationStandardOffsetUnits=m  TranslationStandardAxis=+Z  TranslationCartesianOffset=[0 0 0.5*l]  TranslationCartesianOffsetUnits=m  TranslationROffset=0  TranslationROffsetUnits=m  TranslationZOffset=0  TranslationZOffsetUnits=m  TranslationThetaOffset=0  TranslationThetaOffsetUnits=deg  RotationMethod=AlignedAxes  RotationAngleUnits=deg  RotationStandardAxis=+Z  RotationAngle=0.0  RotationArbitraryAxis=[0 0 1]  FollAlignAxisA=+Z  BaseAlignAxisA=+X  FollAlignAxisB=+Y  BaseAlignAxisB=+Y  RotationSequenceAxes=FollowerAxes  RotationSequence=XYX  RotationSequenceAngles=[0 0 0]  RotationSequenceAnglesUnits=deg  RotationMatrix=[1 0 0; 0 1 0; 0 0 1]  Quaternion=[1 0 0 0]
  Subsystem : Subsystem
  Torsion Joint : sm_lib/Joints/Revolute Joint  JointMode=Normal  SenseConstraintForce=off  SenseConstraintForceX=off  SenseConstraintForceY=off  SenseConstraintForceZ=off  SenseConstraintTorque=off  SenseConstraintTorqueX=off  SenseConstraintTorqueY=off  SenseConstraintTorqueZ=off  SenseTotalForce=off  SenseTotalForceX=off  SenseTotalForceY=off  SenseTotalForceZ=off  SenseTotalTorque=off  SenseTotalTorqueX=off  SenseTotalTorqueY=off  SenseTotalTorqueZ=off  CompositeWrenchDir=FollowerOnBase  CompositeWrenchFrame=BaseFrame  EquilibriumPosition=0  EquilibriumPositionUnits=deg  SpringStiffness=800000  SpringStiffnessUnits=N*m/rad  DampingCoefficient=0  DampingCoefficientUnits=N*m/(deg/s)  TorqueActuationMode=NoTorque  MotionActuationMode=ComputedMotion  SensePosition=on  SenseVelocity=off  SenseAcceleration=off  SenseTorqueForce=off  SenseLowerLimitTorqueForce=off  SenseUpperLimitTorqueForce=off  LowerLimitSpecify=off  LowerLimitBound=-90  LowerLimitBoundUnits=deg  LowerLimitStiffness=1e4  LowerLimitStiffnessUnits=N*m/deg  LowerLimitDamping=10  LowerLimitDampingUnits=N*m/(deg/s)  LowerLimitTransitionRegionWidth=0.1  LowerLimitTransitionRegionWidthUnits=deg  UpperLimitSpecify=off  UpperLimitBound=90  UpperLimitBoundUnits=deg  UpperLimitStiffness=1e4  UpperLimitStiffnessUnits=N*m/deg  UpperLimitDamping=10  UpperLimitDampingUnits=N*m/(deg/s)  UpperLimitTransitionRegionWidth=0.1  UpperLimitTransitionRegionWidthUnits=deg  PositionTargetSpecify=off  PositionTargetPriority=High  PositionTargetValue=0  PositionTargetValueUnits=deg  VelocityTargetSpecify=off  VelocityTargetPriority=High  VelocityTargetValue=0  VelocityTargetValueUnits=deg/s
  Torsion pos : sm_lib/Frames and Transforms/Rigid Transform  TranslationMethod=Cartesian  TranslationStandardOffset=0  TranslationStandardOffsetUnits=m  TranslationStandardAxis=+Z  TranslationCartesianOffset=[(-xcg1+xrev1) 0 0]  TranslationCartesianOffsetUnits=m  TranslationROffset=0  TranslationROffsetUnits=m  TranslationZOffset=0  TranslationZOffsetUnits=m  TranslationThetaOffset=0  TranslationThetaOffsetUnits=deg  RotationMethod=None  RotationAngleUnits=deg  RotationStandardAxis=+Z  RotationAngle=0.0  RotationArbitraryAxis=[0 0 1]  FollAlignAxisA=+X  BaseAlignAxisA=+Y  FollAlignAxisB=+Y  BaseAlignAxisB=+Z  RotationSequenceAxes=FollowerAxes  RotationSequence=XYX  RotationSequenceAngles=[0 0 0]  RotationSequenceAnglesUnits=deg  RotationMatrix=[1 0 0; 0 1 0; 0 0 1]  Quaternion=[1 0 0 0]
  Transform Sensor1 : sm_lib/Frames and Transforms/Transform Sensor  MeasurementFrame=World  RotationSequence=XYX  SenseAngle=off  SenseAxis=off  SenseQ=off  SenseR=on  SenseRotationSequence=off  SenseOmegaX=off  SenseOmegaY=off  SenseOmegaZ=off  SenseQDot=off  SenseRDot=off  SenseRotationSequenceDot=off  SenseAlphaX=off  SenseAlphaY=off  SenseAlphaZ=off  SenseQDDot=off  SenseRDDot=off  SenseX=off  SenseY=off  SenseZ=off  SenseRad=off  SenseAzim=off  SenseDist=off  SenseInc=off  SenseXDot=off  SenseYDot=off  SenseZDot=off  SenseRadDot=off  SenseAzimDot=off  SenseDistDot=off  SenseIncDot=off  SenseXDDot=off  SenseYDDot=off  SenseZDDot=off  SenseRadDDot=off  SenseAzimDDot=off  SenseDistDDot=off  SenseIncDDot=off
  World Frame : sm_lib/Frames and Transforms/World Frame
  Chassis_front : PMIOPort  Side=Left
  Chassis_rear : PMIOPort  Port=2  Side=Right
  Signals : Outport
  signals : Outport  Port=2
  wires:
  PS-Simulink Converter - in rad/1 -> Signals/1
  PS-Simulink Converter4/1 -> Subsystem/1(In1)
  Bus Creator1/1 -> signals/1
  Subsystem/3(roll) -> Bus Creator1/3
  Subsystem/2(pitch) -> Bus Creator1/2
  Subsystem/1(yaw) -> Bus Creator1/1
  connections:
  Torsion pos/LConn1 -- Chassis_front/RConn1
  Chassis rear pos/RConn1 -- Chassis_rear/RConn1
  Realign_Torsion joint/RConn1 -- Chassis rear pos/LConn1
  Align_Torsion joint/RConn1 -- Torsion Joint/LConn1
  Realign_Torsion joint/LConn1 -- Torsion Joint/RConn1
  Align_Torsion joint/LConn1 -- Transform Sensor1/RConn1 -- Torsion pos/RConn1
  Torsion Joint/RConn2 -- PS-Simulink Converter - in rad/LConn1
  PS-Simulink Converter4/LConn1 -- Transform Sensor1/RConn2
  World Frame/RConn1 -- Transform Sensor1/LConn1

== system Tractor_BURGERS_etrailer_v2_1_backup070824/Tractor_semitrailer /To_workspace_semitrailer/Fx Subsystem ==
  In1 : Inport
  Bus Selector24 : BusSelector  OutputSignals=axle1.Tire_L.Longitudinal: Fx,axle1.Tire_R.Longitudinal: Fx,axle2.Tire_L.Longitudinal: Fx,axle2.Tire_R.Longitudinal: Fx,axle3.Tire_L.Longitudinal: Fx,axle3.Tire_R.Longitudinal: Fx
  Mux : Mux  Inputs=6
  Out1 : Outport
  wires:
  In1/1 -> Bus Selector24/1
  Mux/1 -> Out1/1
  Bus Selector24/1 -> Mux/1  "<Longitudinal: Fx>"
  Bus Selector24/2 -> Mux/2  "<Longitudinal: Fx>"
  Bus Selector24/3 -> Mux/3  "<Longitudinal: Fx>"
  Bus Selector24/4 -> Mux/4  "<Longitudinal: Fx>"
  Bus Selector24/5 -> Mux/5  "<Longitudinal: Fx>"
  Bus Selector24/6 -> Mux/6  "<Longitudinal: Fx>"

== system Tractor_BURGERS_etrailer_v2_1_backup070824/Tractor_semitrailer /To_workspace_semitrailer/Fy Subsystem ==
  In1 : Inport
  Bus Selector24 : BusSelector  OutputSignals=axle1.Tire_L.Lateral: Fy,axle1.Tire_R.Lateral: Fy,axle2.Tire_L.Lateral: Fy,axle2.Tire_R.Lateral: Fy,axle3.Tire_L.Lateral: Fy,axle3.Tire_R.Lateral: Fy
  Mux : Mux  Inputs=6
  Out1 : Outport
  wires:
  Bus Selector24/6 -> Mux/6  "<Lateral: Fy>"
  Bus Selector24/5 -> Mux/5  "<Lateral: Fy>"
  Bus Selector24/4 -> Mux/4  "<Lateral: Fy>"
  Bus Selector24/3 -> Mux/3  "<Lateral: Fy>"
  Bus Selector24/2 -> Mux/2  "<Lateral: Fy>"
  Bus Selector24/1 -> Mux/1  "<Lateral: Fy>"
  In1/1 -> Bus Selector24/1
  Mux/1 -> Out1/1

== system Tractor_BURGERS_etrailer_v2_1_backup070824/Tractor_semitrailer /To_workspace_semitrailer/Fz Subsystem ==
  In1 : Inport
  Bus Selector24 : BusSelector  OutputSignals=axle1.Tire_L.Normal: Fz,axle1.Tire_R.Normal: Fz,axle2.Tire_L.Normal: Fz,axle2.Tire_R.Normal: Fz,axle3.Tire_L.Normal: Fz,axle3.Tire_R.Normal: Fz
  Mux : Mux  Inputs=6
  Out1 : Outport
  wires:
  Mux/1 -> Out1/1
  In1/1 -> Bus Selector24/1
  Bus Selector24/1 -> Mux/1  "<Normal: Fz>"
  Bus Selector24/2 -> Mux/2  "<Normal: Fz>"
  Bus Selector24/3 -> Mux/3  "<Normal: Fz>"
  Bus Selector24/4 -> Mux/4  "<Normal: Fz>"
  Bus Selector24/5 -> Mux/5  "<Normal: Fz>"
  Bus Selector24/6 -> Mux/6  "<Normal: Fz>"

== system Tractor_BURGERS_etrailer_v2_1_backup070824/Tractor_semitrailer /To_workspace_semitrailer/Mz Subsystem ==
  In1 : Inport
  Bus Selector24 : BusSelector  OutputSignals=axle1.Tire_L.Aligning: Mz,axle1.Tire_R.Aligning: Mz,axle2.Tire_L.Aligning: Mz,axle2.Tire_R.Aligning: Mz,axle3.Tire_L.Aligning: Mz,axle3.Tire_R.Aligning: Mz
  Mux : Mux  Inputs=6
  Out1 : Outport
  wires:
  Mux/1 -> Out1/1
  In1/1 -> Bus Selector24/1
  Bus Selector24/1 -> Mux/1  "<Aligning: Mz>"
  Bus Selector24/2 -> Mux/2  "<Aligning: Mz>"
  Bus Selector24/3 -> Mux/3  "<Aligning: Mz>"
  Bus Selector24/4 -> Mux/4  "<Aligning: Mz>"
  Bus Selector24/5 -> Mux/5  "<Aligning: Mz>"
  Bus Selector24/6 -> Mux/6  "<Aligning: Mz>"

== system Tractor_BURGERS_etrailer_v2_1_backup070824/Tractor_semitrailer /To_workspace_semitrailer/Omega Subsystem ==
  In1 : Inport
  Bus Selector6 : BusSelector  OutputSignals=axle1.Omega1,axle1.Omega2,axle2.Omega1,axle2.Omega2,axle3.Omega1,axle3.Omega2
  Mux : Mux  Inputs=6
  Out1 : Outport
  wires:
  Bus Selector6/6 -> Mux/6  "<Omega2>"
  Bus Selector6/5 -> Mux/5  "<Omega1>"
  Bus Selector6/4 -> Mux/4  "<Omega2>"
  Bus Selector6/3 -> Mux/3  "<Omega1>"
  Bus Selector6/2 -> Mux/2  "<Omega2>"
  Bus Selector6/1 -> Mux/1  "<Omega1>"
  Mux/1 -> Out1/1
  In1/1 -> Bus Selector6/1

== system Tractor_BURGERS_etrailer_v2_1_backup070824/Tractor_semitrailer /To_workspace_tractor/Fx Subsystem ==
  In : Inport
  Bus Selector24 : BusSelector  OutputSignals=steeraxle.Tire1_L.Longitudinal: Fx,steeraxle.Tire1_R.Longitudinal: Fx,driveaxle.Tire1_L.Longitudinal: Fx,driveaxle.Tire1_R.Longitudinal: Fx,driveaxle.Tire2_L.Longitudinal: Fx,driveaxle.Tire2_R.Longitudinal: Fx
  Mux : Mux  Inputs=6
  Out : Outport
  wires:
  In/1 -> Bus Selector24/1
  Mux/1 -> Out/1
  Bus Selector24/1 -> Mux/1  "<Longitudinal: Fx>"
  Bus Selector24/2 -> Mux/2  "<Longitudinal: Fx>"
  Bus Selector24/3 -> Mux/3  "<Longitudinal: Fx>"
  Bus Selector24/4 -> Mux/4  "<Longitudinal: Fx>"
  Bus Selector24/5 -> Mux/5  "<Longitudinal: Fx>"
  Bus Selector24/6 -> Mux/6  "<Longitudinal: Fx>"

== system Tractor_BURGERS_etrailer_v2_1_backup070824/Tractor_semitrailer /To_workspace_tractor/Fy Subsystem ==
  In1 : Inport
  Bus Selector24 : BusSelector  OutputSignals=steeraxle.Tire1_L.Lateral: Fy,steeraxle.Tire1_R.Lateral: Fy,driveaxle.Tire1_L.Lateral: Fy,driveaxle.Tire1_R.Lateral: Fy,driveaxle.Tire2_L.Lateral: Fy,driveaxle.Tire2_R.Lateral: Fy
  Mux : Mux  Inputs=6
  Out1 : Outport
  wires:
  In1/1 -> Bus Selector24/1
  Mux/1 -> Out1/1
  Bus Selector24/1 -> Mux/1  "<Lateral: Fy>"
  Bus Selector24/2 -> Mux/2  "<Lateral: Fy>"
  Bus Selector24/3 -> Mux/3  "<Lateral: Fy>"
  Bus Selector24/4 -> Mux/4  "<Lateral: Fy>"
  Bus Selector24/5 -> Mux/5  "<Lateral: Fy>"
  Bus Selector24/6 -> Mux/6  "<Lateral: Fy>"

== system Tractor_BURGERS_etrailer_v2_1_backup070824/Tractor_semitrailer /To_workspace_tractor/Fz Subsystem ==
  In1 : Inport
  Bus Selector24 : BusSelector  OutputSignals=steeraxle.Tire1_L.Normal: Fz,steeraxle.Tire1_R.Normal: Fz,driveaxle.Tire1_L.Normal: Fz,driveaxle.Tire1_R.Normal: Fz,driveaxle.Tire2_L.Normal: Fz,driveaxle.Tire2_R.Normal: Fz
  Mux : Mux  Inputs=6
  Out1 : Outport
  wires:
  In1/1 -> Bus Selector24/1
  Mux/1 -> Out1/1
  Bus Selector24/1 -> Mux/1  "<Normal: Fz>"
  Bus Selector24/2 -> Mux/2  "<Normal: Fz>"
  Bus Selector24/3 -> Mux/3  "<Normal: Fz>"
  Bus Selector24/4 -> Mux/4  "<Normal: Fz>"
  Bus Selector24/5 -> Mux/5  "<Normal: Fz>"
  Bus Selector24/6 -> Mux/6  "<Normal: Fz>"

== system Tractor_BURGERS_etrailer_v2_1_backup070824/Tractor_semitrailer /To_workspace_tractor/Mz Subsystem ==
  In1 : Inport
  Bus Selector24 : BusSelector  OutputSignals=steeraxle.Tire1_L.Aligning: Mz,steeraxle.Tire1_R.Aligning: Mz,driveaxle.Tire1_L.Aligning: Mz,driveaxle.Tire1_R.Aligning: Mz,driveaxle.Tire2_L.Aligning: Mz,driveaxle.Tire2_R.Aligning: Mz
  Mux : Mux  Inputs=6
  Out1 : Outport
  wires:
  In1/1 -> Bus Selector24/1
  Bus Selector24/6 -> Mux/6  "<Aligning: Mz>"
  Mux/1 -> Out1/1
  Bus Selector24/5 -> Mux/5  "<Aligning: Mz>"
  Bus Selector24/1 -> Mux/1  "<Aligning: Mz>"
  Bus Selector24/3 -> Mux/3  "<Aligning: Mz>"
  Bus Selector24/4 -> Mux/4  "<Aligning: Mz>"
  Bus Selector24/2 -> Mux/2  "<Aligning: Mz>"

== system Tractor_BURGERS_etrailer_v2_1_backup070824/Tractor_semitrailer /To_workspace_tractor/Omega Subsystem ==
  In1 : Inport
  Bus Selector6 : BusSelector  OutputSignals=steeraxle.Omega1,steeraxle.Omega2,driveaxle.Omega1,driveaxle.Omega2
  Mux : Mux
  Out1 : Outport
  wires:
  Bus Selector6/2 -> Mux/2  "<Omega2>"
  Bus Selector6/4 -> Mux/4  "<Omega2>"
  Bus Selector6/3 -> Mux/3  "<Omega1>"
  Bus Selector6/1 -> Mux/1  "<Omega1>"
  Mux/1 -> Out1/1
  In1/1 -> Bus Selector6/1

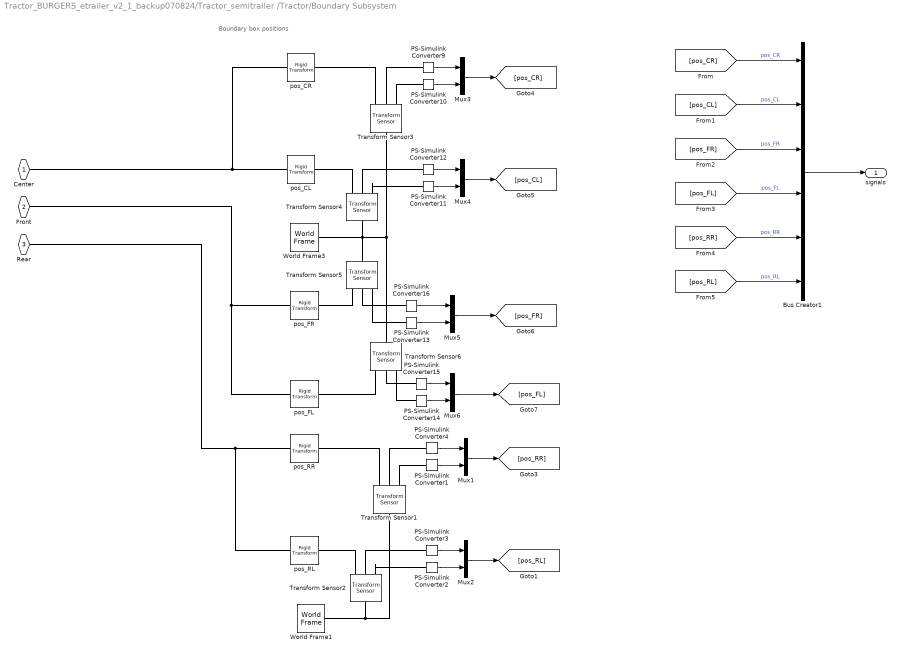
== system Tractor_BURGERS_etrailer_v2_1_backup070824/Tractor_semitrailer /Tractor/Boundary Subsystem ==
  note: Boundary box positions
  Bus Creator1 : BusCreator  Inputs=6
  Mux{1..6} (6 alike) : Mux  Inputs=2
  PS-Simulink Converter{1..4,9..16} (12 alike) : nesl_utility/PS-Simulink Converter  PhysicalDomain=network_engine_domain  SubClassName=ps_output  LeftPortType=input  RightPortType=output  PseudoPeriodic=off  Frequencies=[]  VectorFormat=1-D array  Unit=inherit  AffineConversion=off
  Transform Sensor{1..6} (6 alike) : sm_lib/Frames and Transforms/Transform Sensor  MeasurementFrame=World  RotationSequence=XYX  SenseAngle=off  SenseAxis=off  SenseQ=off  SenseR=off  SenseRotationSequence=off  SenseOmegaX=off  SenseOmegaY=off  SenseOmegaZ=off  SenseQDot=off  SenseRDot=off  SenseRotationSequenceDot=off  SenseAlphaX=off  SenseAlphaY=off  SenseAlphaZ=off  SenseQDDot=off  SenseRDDot=off  SenseX=on  SenseY=on  SenseZ=off  SenseRad=off  SenseAzim=off  SenseDist=off  SenseInc=off  SenseXDot=off  SenseYDot=off  SenseZDot=off  SenseRadDot=off  SenseAzimDot=off  SenseDistDot=off  SenseIncDot=off  SenseXDDot=off  SenseYDDot=off  SenseZDDot=off  SenseRadDDot=off  SenseAzimDDot=off  SenseDistDDot=off  SenseIncDDot=off
  World Frame1 : sm_lib/Frames and Transforms/World Frame
  World Frame3 : sm_lib/Frames and Transforms/World Frame
  pos_CL : sm_lib/Frames and Transforms/Rigid Transform  TranslationMethod=Cartesian  TranslationStandardOffset=0  TranslationStandardOffsetUnits=m  TranslationStandardAxis=+Z  TranslationCartesianOffset=[0 1.25 -h1/2]  TranslationCartesianOffsetUnits=m  TranslationROffset=0  TranslationROffsetUnits=m  TranslationZOffset=0  TranslationZOffsetUnits=m  TranslationThetaOffset=0  TranslationThetaOffsetUnits=deg  RotationMethod=None  RotationAngleUnits=deg  RotationStandardAxis=+Z  RotationAngle=0.0  RotationArbitraryAxis=[0 0 1]  FollAlignAxisA=+X  BaseAlignAxisA=+Y  FollAlignAxisB=+Y  BaseAlignAxisB=+Z  RotationSequenceAxes=FollowerAxes  RotationSequence=XYX  RotationSequenceAngles=[0 0 0]  RotationSequenceAnglesUnits=deg  RotationMatrix=[1 0 0; 0 1 0; 0 0 1]  Quaternion=[1 0 0 0]
  pos_CR : sm_lib/Frames and Transforms/Rigid Transform  TranslationMethod=Cartesian  TranslationStandardOffset=0  TranslationStandardOffsetUnits=m  TranslationStandardAxis=+Z  TranslationCartesianOffset=[0 -1.25 -h1/2]  TranslationCartesianOffsetUnits=m  TranslationROffset=0  TranslationROffsetUnits=m  TranslationZOffset=0  TranslationZOffsetUnits=m  TranslationThetaOffset=0  TranslationThetaOffsetUnits=deg  RotationMethod=None  RotationAngleUnits=deg  RotationStandardAxis=+Z  RotationAngle=0.0  RotationArbitraryAxis=[0 0 1]  FollAlignAxisA=+X  BaseAlignAxisA=+Y  FollAlignAxisB=+Y  BaseAlignAxisB=+Z  RotationSequenceAxes=FollowerAxes  RotationSequence=XYX  RotationSequenceAngles=[0 0 0]  RotationSequenceAnglesUnits=deg  RotationMatrix=[1 0 0; 0 1 0; 0 0 1]  Quaternion=[1 0 0 0]
  pos_FL : sm_lib/Frames and Transforms/Rigid Transform  TranslationMethod=Cartesian  TranslationStandardOffset=0  TranslationStandardOffsetUnits=m  TranslationStandardAxis=+Z  TranslationCartesianOffset=[0 1.25 -h1/2]  TranslationCartesianOffsetUnits=m  TranslationROffset=0  TranslationROffsetUnits=m  TranslationZOffset=0  TranslationZOffsetUnits=m  TranslationThetaOffset=0  TranslationThetaOffsetUnits=deg  RotationMethod=None  RotationAngleUnits=deg  RotationStandardAxis=+Z  RotationAngle=0.0  RotationArbitraryAxis=[0 0 1]  FollAlignAxisA=+X  BaseAlignAxisA=+Y  FollAlignAxisB=+Y  BaseAlignAxisB=+Z  RotationSequenceAxes=FollowerAxes  RotationSequence=XYX  RotationSequenceAngles=[0 0 0]  RotationSequenceAnglesUnits=deg  RotationMatrix=[1 0 0; 0 1 0; 0 0 1]  Quaternion=[1 0 0 0]
  pos_FR : sm_lib/Frames and Transforms/Rigid Transform  TranslationMethod=Cartesian  TranslationStandardOffset=0  TranslationStandardOffsetUnits=m  TranslationStandardAxis=+Z  TranslationCartesianOffset=[0 -1.25 -h1/2]  TranslationCartesianOffsetUnits=m  TranslationROffset=0  TranslationROffsetUnits=m  TranslationZOffset=0  TranslationZOffsetUnits=m  TranslationThetaOffset=0  TranslationThetaOffsetUnits=deg  RotationMethod=None  RotationAngleUnits=deg  RotationStandardAxis=+Z  RotationAngle=0.0  RotationArbitraryAxis=[0 0 1]  FollAlignAxisA=+X  BaseAlignAxisA=+Y  FollAlignAxisB=+Y  BaseAlignAxisB=+Z  RotationSequenceAxes=FollowerAxes  RotationSequence=XYX  RotationSequenceAngles=[0 0 0]  RotationSequenceAnglesUnits=deg  RotationMatrix=[1 0 0; 0 1 0; 0 0 1]  Quaternion=[1 0 0 0]
  pos_RL : sm_lib/Frames and Transforms/Rigid Transform  TranslationMethod=Cartesian  TranslationStandardOffset=0  TranslationStandardOffsetUnits=m  TranslationStandardAxis=+Z  TranslationCartesianOffset=[0 1.25 -h2/2]  TranslationCartesianOffsetUnits=m  TranslationROffset=0  TranslationROffsetUnits=m  TranslationZOffset=0  TranslationZOffsetUnits=m  TranslationThetaOffset=0  TranslationThetaOffsetUnits=deg  RotationMethod=None  RotationAngleUnits=deg  RotationStandardAxis=+Z  RotationAngle=0.0  RotationArbitraryAxis=[0 0 1]  FollAlignAxisA=+X  BaseAlignAxisA=+Y  FollAlignAxisB=+Y  BaseAlignAxisB=+Z  RotationSequenceAxes=FollowerAxes  RotationSequence=XYX  RotationSequenceAngles=[0 0 0]  RotationSequenceAnglesUnits=deg  RotationMatrix=[1 0 0; 0 1 0; 0 0 1]  Quaternion=[1 0 0 0]
  pos_RR : sm_lib/Frames and Transforms/Rigid Transform  TranslationMethod=Cartesian  TranslationStandardOffset=0  TranslationStandardOffsetUnits=m  TranslationStandardAxis=+Z  TranslationCartesianOffset=[0 -1.25 -h2/2]  TranslationCartesianOffsetUnits=m  TranslationROffset=0  TranslationROffsetUnits=m  TranslationZOffset=0  TranslationZOffsetUnits=m  TranslationThetaOffset=0  TranslationThetaOffsetUnits=deg  RotationMethod=None  RotationAngleUnits=deg  RotationStandardAxis=+Z  RotationAngle=0.0  RotationArbitraryAxis=[0 0 1]  FollAlignAxisA=+X  BaseAlignAxisA=+Y  FollAlignAxisB=+Y  BaseAlignAxisB=+Z  RotationSequenceAxes=FollowerAxes  RotationSequence=XYX  RotationSequenceAngles=[0 0 0]  RotationSequenceAnglesUnits=deg  RotationMatrix=[1 0 0; 0 1 0; 0 0 1]  Quaternion=[1 0 0 0]
  Center : PMIOPort  Side=Right
  Front : PMIOPort  Port=2  Side=Right
  Rear : PMIOPort  Port=3  Side=Right
  signals : Outport
  wires:
  PS-Simulink Converter13/1 -> Mux5/2
  PS-Simulink Converter10/1 -> Mux3/2
  PS-Simulink Converter16/1 -> Mux5/1
  Mux6/1 -> [pos_FL]
  PS-Simulink Converter15/1 -> Mux6/1
  PS-Simulink Converter14/1 -> Mux6/2
  Mux5/1 -> [pos_FR]
  PS-Simulink Converter9/1 -> Mux3/1
  Mux3/1 -> [pos_CR]
  PS-Simulink Converter11/1 -> Mux4/2
  PS-Simulink Converter12/1 -> Mux4/1
  Mux4/1 -> [pos_CL]
  PS-Simulink Converter1/1 -> Mux1/2
  Mux2/1 -> [pos_RL]
  Mux1/1 -> [pos_RR]
  PS-Simulink Converter3/1 -> Mux2/1
  PS-Simulink Converter2/1 -> Mux2/2
  PS-Simulink Converter4/1 -> Mux1/1
  [pos_RL] -> Bus Creator1/6  "pos_RL"
  [pos_RR] -> Bus Creator1/5  "pos_RR"
  [pos_FL] -> Bus Creator1/4  "pos_FL"
  [pos_FR] -> Bus Creator1/3  "pos_FR"
  [pos_CL] -> Bus Creator1/2  "pos_CL"
  [pos_CR] -> Bus Creator1/1  "pos_CR"
  Bus Creator1/1 -> signals/1
  connections:
  Transform Sensor6/LConn1 -- Transform Sensor3/LConn1 -- Transform Sensor5/LConn1 -- Transform Sensor4/LConn1 -- World Frame3/RConn1
  pos_FR/LConn1 -- Front/RConn1 -- pos_FL/LConn1
  pos_CL/LConn1 -- Center/RConn1 -- pos_CR/LConn1
  Transform Sensor3/RConn1 -- pos_CR/RConn1
  Transform Sensor5/RConn1 -- pos_FR/RConn1
  Transform Sensor6/RConn1 -- pos_FL/RConn1
  Transform Sensor4/RConn3 -- PS-Simulink Converter11/LConn1
  Transform Sensor4/RConn2 -- PS-Simulink Converter12/LConn1
  Transform Sensor5/RConn2 -- PS-Simulink Converter16/LConn1
  Transform Sensor6/RConn3 -- PS-Simulink Converter14/LConn1
  Transform Sensor6/RConn2 -- PS-Simulink Converter15/LConn1
  Transform Sensor3/RConn3 -- PS-Simulink Converter10/LConn1
  Transform Sensor3/RConn2 -- PS-Simulink Converter9/LConn1
  Transform Sensor5/RConn3 -- PS-Simulink Converter13/LConn1
  Transform Sensor4/RConn1 -- pos_CL/RConn1
  pos_RL/LConn1 -- Rear/RConn1 -- pos_RR/LConn1
  Transform Sensor1/LConn1 -- Transform Sensor2/LConn1 -- World Frame1/RConn1
  Transform Sensor2/RConn1 -- pos_RL/RConn1
  Transform Sensor1/RConn1 -- pos_RR/RConn1
  Transform Sensor2/RConn2 -- PS-Simulink Converter3/LConn1
  Transform Sensor1/RConn2 -- PS-Simulink Converter4/LConn1
  Transform Sensor1/RConn3 -- PS-Simulink Converter1/LConn1
  Transform Sensor2/RConn3 -- PS-Simulink Converter2/LConn1
